simulink model "Doublet"  (R2021a)
settings: Solver=VariableStepAuto  StartTime=0.0  StopTime=10.0  RelTol=1e-3
settings Model: Creator=Camden  LastModifiedBy=Camden
settings SolverCC: AlgebraicLoopSolver=TrustRegion
settings DebuggingCC: SFMachineParentedDataDiag=warning

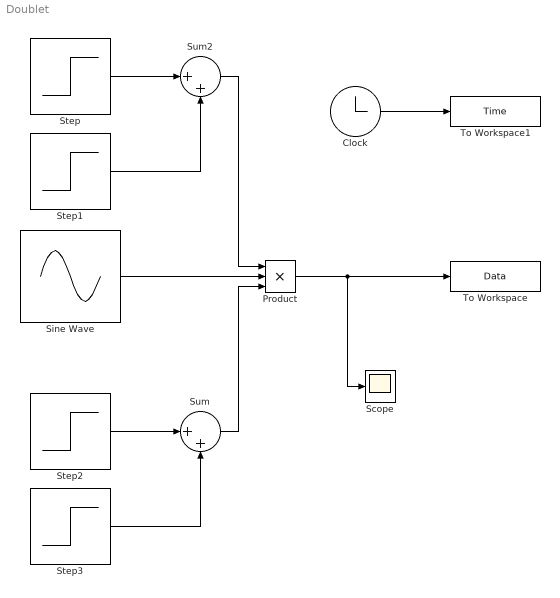
== system Doublet ==
  Clock : Clock
  Product : Product  Inputs=3
  Scope : Scope
  Sine Wave : Sin  Amplitude=1.000  Frequency=.5*(2*pi)  SampleTime=0
  Step : Step  Time=0  After=0  SampleTime=0
  Step1 : Step  Time=2  SampleTime=0
  Step2 : Step  Time=4  Before=1  After=0  SampleTime=0
  Step3 : Step  Time=6  After=0  SampleTime=0
  Sum : Sum  Inputs=|++
  Sum2 : Sum  Inputs=|++
  To Workspace : ToWorkspace  VariableName=Data  SaveFormat=Timeseries  SampleTime=-1
  To Workspace1 : ToWorkspace  VariableName=Time  SaveFormat=Timeseries  SampleTime=-1
  wires:
  Sine Wave/1 -> Product/2
  Step1/1 -> Sum2/2
  Step/1 -> Sum2/1
  Sum2/1 -> Product/1
  Step2/1 -> Sum/1
  Step3/1 -> Sum/2
  Sum/1 -> Product/3
  Product/1 -> Scope/1, To Workspace/1
  Clock/1 -> To Workspace1/1
